simulink model "SetReset_tmp"  (Simulink 8.3)
settings: Solver=FixedStepDiscrete  StartTime=0.0  StopTime=inf  RelTol=1e-3
settings Model: Creator=scaife  LastModifiedBy=hbourbou  CovSFcnEnable=on  ExtModeAutoUpdateStatusClock=off
settings DataIOCC: SignalLoggingName=sigsOut
settings OptimizationCC: InitFltsAndDblsToZero=on
settings DebuggingCC: SaveWithParameterizedLinksMsg=none  SignalResolutionControl=TryResolveAllWithWarning  SolverPrmCheckMsg=none  MultiTaskDSMMsg=warning  MultiTaskCondExecSysMsg=none  FrameProcessingCompatibilityMsg=error  StateNameClashWarn=none  StrictBusMsg=None
settings HardwareCC: TargetUnknown=on
settings SFSimCC: SimParseCustomCode=off
settings GRTTargetCC: TargetFcnLib=ansi_tfl_tmw.mat  ModelReferenceCompliant=off  GeneratePreprocessorConditionals=Use local settings  MatFileLogging=off

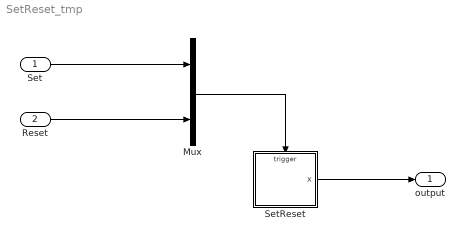
== system SetReset_tmp ==
  Set : Inport
  Reset : Inport  Port=2
  Mux : Mux  Inputs=2
  SetReset : Stateflow chart  TreatAsAtomicUnit=on
      settings: PermitHierarchicalResolution=ParametersOnly
  output : Outport
  wires:
  Mux/1 -> SetReset/Trigger
  Set/1 -> Mux/1
  Reset/1 -> Mux/2
  SetReset/1(x) -> output/1

== stateflow chart SetReset ==
  state Off/
    en:x=0
  state On/
    en:x=1
  (default) -> Off
  Off -> On : Set
  On -> Off : Reset
  data: x output int32
  events: Set input RISING_EDGE_EVENT; Reset input RISING_EDGE_EVENT
